simulink model "vehicle_start"  (R2018a)
settings: Solver=ode45  StartTime=0.0  StopTime=10  RelTol=1e-3  EnableMultiTasking=on
PreLoadFcn:
  | m = 104.2;
  | Cd = 0.4;
  | rho = 2.377e-3;
  | h = 4.15;
  | w = 5.71;
settings Model: Creator=jrivitus  LastModifiedBy=bneiswan
settings DataIOCC: LimitDataPoints=on  SaveFormat=Array
settings OptimizationCC: ExpressionDepthLimit=2147483647  LifeSpan=inf
settings DebuggingCC: UnderspecifiedInitializationDetection=Classic  MergeDetectMultiDrivingBlocksExec=none  ParameterPrecisionLossMsg=none  FcnCallInpInsideContextMsg=warning  AllowSymbolicDim=off  StateNameClashWarn=warning  SFUnexpectedBacktrackingDiag=warning  SFNoUnconditionalDefaultTransitionDiag=warning  SFExecutionAtInitializationDiag=none
settings HardwareCC: ProdBitPerPointer=32  ProdBitPerSizeT=32  ProdBitPerPtrDiffT=32  ProdLargestAtomicFloat=None  ProdIntDivRoundTo=Undefined  ProdEndianess=Unspecified  ProdWordSize=32  ProdHWDeviceType=32-bit Generic
settings ModelReferenceCC: PropagateSignalLabelsOutOfModel=off
settings CodeAppCC: StateflowObjectComments=on
settings GRTTargetCC: TargetLangStandard=C89/C90 (ANSI)  GeneratePreprocessorConditionals=Disable all  CombineOutputUpdateFcns=off  GRTInterface=on
settings ConfigComp: CovMetricSettings=dw  CovHtmlReporting=on  CovSaveCumulativeToWorkspaceVar=on  CovSaveSingleToWorkspaceVar=on  CovExternalEMLEnable=off  CovSFcnEnable=off

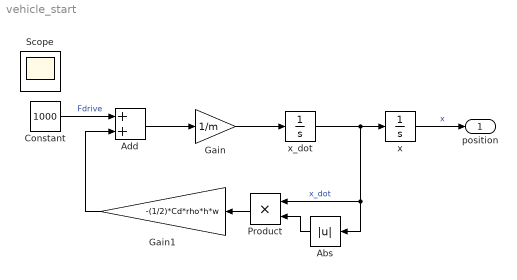
== system vehicle_start ==
  Abs : Abs
  Add : Sum
  Constant : Constant  Value=1000
  Gain : Gain  Gain=1/m
  Gain1 : Gain  Gain=-(1/2)*Cd*rho*h*w
  Product : Product  RndMeth=Zero
  x : Integrator
  x_dot : Integrator
  position : Outport
  Scope : Scope
  wires:
  Constant/1 -> Add/1  "Fdrive"
  x_dot/1 -> x/1, Product/1, Abs/1  "x_dot"
  x/1 -> position/1  "x"
  Add/1 -> Gain/1
  Gain/1 -> x_dot/1
  Abs/1 -> Product/2
  Product/1 -> Gain1/1
  Gain1/1 -> Add/2
